simulink library "SpikingLib"  (Simulink 7.5)
settings: Solver=ode45  SolverMode=SingleTasking  StartTime=0.0  StopTime=10.0  RelTol=1e-3
undefined symbols (not defined in the file or in its folder): windowDuration
libraries: SpikingLib x13, simulink x3
settings Model: Creator=jpalma  LastModifiedBy=jpalma

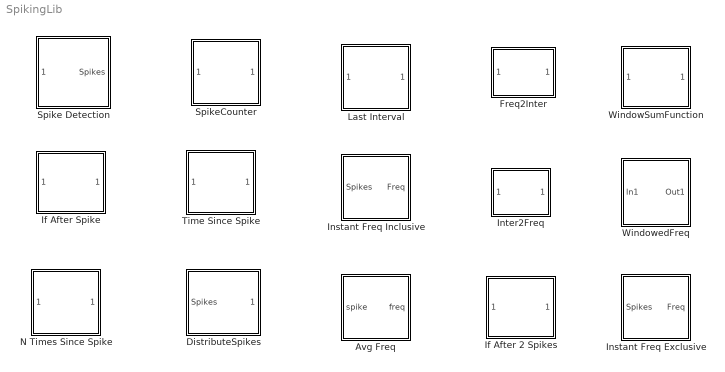
== system SpikingLib ==
  Avg Freq : Subsystem
      mask Description: Author: Jesse Palma
      mask Help: Author: Jesse Palma
      mask Display: image(imread('../Libs/icons/AvgFreq.jpg'),'center');
  DistributeSpikes : Subsystem  mask{numChannels=3}
      mask prompts: numChannels "Number of Channels"
      mask help:
      | Does not work with vectors of spike trains.
      |
      | Author: Jesse Palma
      mask Help: Author: Jesse Palma
      mask Display: image(imread('../Libs/icons/DistribSpikes.jpg'),'center');
  Freq2Inter : Subsystem
      mask Description: Author: Jesse Palma
      mask Help: Author: Jesse Palma
      mask Display: image(imread('../Libs/icons/FreqInter.jpg'),'center');
  If After 2 Spikes : Subsystem
      mask Description:
      | Are we after the second spike?
      | 
      | With an input vector of spike trains, this produces a vector of booleans of whether 2 spikes have arrived.
      | 
      | Author: Jesse Palma
      mask Help: Author: Jesse Palma
      mask Display: image(imread('../Libs/icons/IfAfterSpike.jpg'), 'center');
  If After Spike : Subsystem
      mask Description:
      | Are we after the first spike?
      | 
      | With an input vector of spike trains, this produces a vector of booleans of whether first spike has arrived.
      | 
      | Author: Jesse Palma
      mask Help: Author: Jesse Palma
      mask Display: image(imread('../Libs/icons/IfAfterSpike.jpg'), 'center');
  Instant Freq Exclusive : Subsystem
      mask Description:
      | Calculates frequency as 1 over the last interspike interval.
      | Frequency therefore isn't calculated until after the 2nd spike.
      | 
      | Author: Jesse Palma
      mask Help:
      | Calculates frequency as 1 over the last interspike interval.
      | Frequency therefore isn't calculated until after the 2nd spike.
      | 
      | Author: Jesse Palma
      mask Display: image(imread('../Libs/icons/InstantFreq.jpg'),'center');
  Instant Freq Inclusive : Subsystem
      mask Description:
      | Calculates frequency as 1 over the last interspike interval or the simulation time over first spike.
      | 
      | Author: Jesse Palma
      mask Help:
      | Calculates frequency as 1 over the last interspike interval or the simulation time over first spike.
      | 
      | Author: Jesse Palma
      mask Display: image(imread('../Libs/icons/InstantFreq.jpg'),'center');
  Inter2Freq : Subsystem
      mask Description: Author: Jesse Palma
      mask Help: Author: Jesse Palma
      mask Display: image(imread('../Libs/icons/InterFreq.jpg'),'center');
  Last Interval : Subsystem
      mask Description:
      | How long was the last interval?
      | 
      | With an input vector of spike trains, this produces a vector of last interspike interval durations.
      | 
      | Author: Jesse Palma
      mask Help: Author: Jesse Palma
      mask Display: image(imread('../Libs/icons/LastInterval.jpg'),'center');
  N Times Since Spike : Subsystem  mask{spikesMemory=10}
      mask prompts: spikesMemory "Size of Spikes Memory"
      mask help:
      | Does not work with vectors of spike trains.
      |
      | Author: Jesse Palma
      mask Help: Author: Jesse Palma
      mask Display: image(imread('../Libs/icons/NTimeSinceSpike.jpg'),'center');
  Spike Detection : Subsystem  mask{SpikeVoltageThreshold=10}
      mask prompts: SpikeVoltageThreshold "Spike Voltage Threshold"
      mask help: Author: Jesse Palma
      mask Help: Author: Jesse Palma
      mask Display: image(imread('../Libs/icons/SpikeDetection.jpg'),'center');
  SpikeCounter : Subsystem
      mask Description:
      | How many spikes so far?
      | 
      | With an input vector of spike trains, this produces a vector of the number of spikes arrived.
      | 
      | Author: Jesse Palma
      mask Help: Author: Jesse Palma
      mask Display: image(imread('../Libs/icons/SpikeCounter.jpg'),'center');
  Time Since Spike : Subsystem
      mask Description:
      | How long since the last spike?
      | 
      | With an input vector of spike trains, this produces a vector of times since the last spike arrived.
      | 
      | Author: Jesse Palma
      mask Help: Author: Jesse Palma
      mask Display: image(imread('../Libs/icons/TimeSinceSpike.jpg'),'center');
  WindowSumFunction : Subsystem  mask{windowDuration=windowDuration}
      mask prompts: windowDuration "Window Duration"
      mask help: Author: Jesse Palma
      mask Help: Author: Jesse Palma
      mask Display: image(imread('../Libs/icons/SquareWave.jpg'),'center');
  WindowedFreq : Subsystem  mask{windowDuration=60, spikesMemory=15}
      mask prompts: windowDuration "Window Duration"; spikesMemory "Max Number of Spikes Stored"
      mask help:
      | Note:
      |   maxFreq = spikesStored*1000/windowDuration
      |   freqPrecision = 1000/windowDuration
      | e.g. Defaults
      |   maxFreq = 15*1000/60 = 250
      |   freqPrecision = 1000/60 = 18
      |
      | Does not work with vectors of spike trains.
      |
      | Author: Jesse Palma
      mask Help: Author: Jesse Palma
      mask Display: image(imread('../Libs/icons/WindFreq.jpg'),'center');

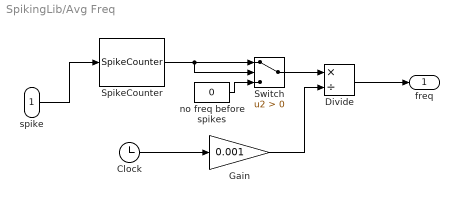
== system SpikingLib/Avg Freq ==
  spike : Inport
  Clock : Clock
      settings: Decimation=10
  Divide : Product  Inputs=*/
  Gain : Gain  Gain=0.001
  SpikeCounter : SpikingLib/SpikeCounter  SystemSampleTime=-1
  Switch : Switch  Criteria=u2 > Threshold
  no freq before spikes : Constant  Value=0
  freq : Outport
  wires:
  Divide/1 -> freq/1
  spike/1 -> SpikeCounter/1
  Clock/1 -> Gain/1
  Gain/1 -> Divide/2
  no freq before spikes/1 -> Switch/3
  Switch/1 -> Divide/1
  SpikeCounter/1 -> Switch/2, Switch/1

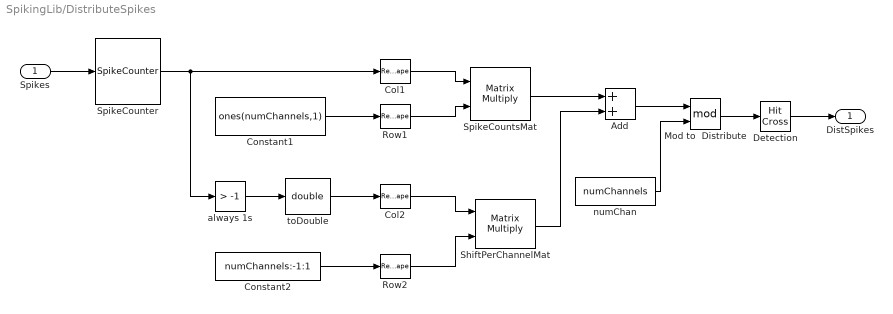
== system SpikingLib/DistributeSpikes ==
  Spikes : Inport
  Add : Sum
  Col1 : Reshape  OutputDimensionality=Column vector (2-D)
  Col2 : Reshape  OutputDimensionality=Column vector (2-D)
  Constant1 : Constant  Value=ones(numChannels,1)
  Constant2 : Constant  Value=numChannels:-1:1
  Detection : HitCross  HitCrossingDirection=rising
  Mod to  Distribute : Math  Operator=mod  SaturateOnIntegerOverflow=on
  Row1 : Reshape  OutputDimensionality=Row vector (2-D)
  Row2 : Reshape  OutputDimensionality=Row vector (2-D)
  ShiftPerChannelMat : Product  Multiplication=Matrix(*)  RndMeth=Zero
  SpikeCounter : SpikingLib/SpikeCounter  SystemSampleTime=-1
  SpikeCountsMat : Product  Multiplication=Matrix(*)  RndMeth=Zero
  always 1s : simulink/Logic and Bit Operations/Compare To Constant  SystemSampleTime=-1  relop=>  const=-1  LogicOutDataTypeMode=uint8  ZeroCross=off
  numChan : Constant  Value=numChannels
  toDouble : DataTypeConversion  OutDataTypeMode=double  OutDataTypeStr=double
  DistSpikes : Outport
  wires:
  SpikeCounter/1 -> always 1s/1, Col1/1
  numChan/1 -> Mod to  Distribute/2
  Mod to  Distribute/1 -> Detection/1
  Col1/1 -> SpikeCountsMat/1
  Constant1/1 -> Row1/1
  Constant2/1 -> Row2/1
  always 1s/1 -> toDouble/1
  toDouble/1 -> Col2/1
  Row2/1 -> ShiftPerChannelMat/2
  SpikeCountsMat/1 -> Add/1
  ShiftPerChannelMat/1 -> Add/2
  Add/1 -> Mod to  Distribute/1
  Spikes/1 -> SpikeCounter/1
  Detection/1 -> DistSpikes/1
  Col2/1 -> ShiftPerChannelMat/1
  Row1/1 -> SpikeCountsMat/2

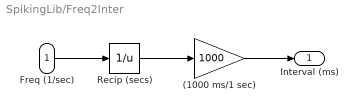
== system SpikingLib/Freq2Inter ==
  Freq (1/sec) : Inport
  (1000 ms/1 sec) : Gain  Gain=1000
  Recip (secs) : Math  Operator=reciprocal  SaturateOnIntegerOverflow=on
  Interval (ms) : Outport
  wires:
  (1000 ms/1 sec)/1 -> Interval (ms)/1
  Freq (1/sec)/1 -> Recip (secs)/1
  Recip (secs)/1 -> (1000 ms/1 sec)/1

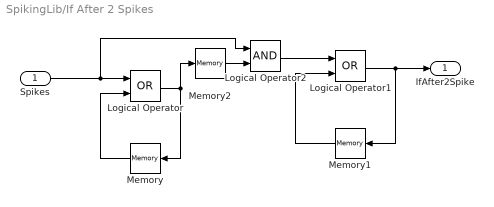
== system SpikingLib/If After 2 Spikes ==
  Spikes : Inport
  Logical Operator : Logic  Operator=OR  AllPortsSameDT=off  OutDataTypeMode=boolean  OutDataTypeStr=boolean
  Logical Operator1 : Logic  Operator=OR  AllPortsSameDT=off  OutDataTypeMode=boolean  OutDataTypeStr=boolean
  Logical Operator2 : Logic  AllPortsSameDT=off  OutDataTypeMode=boolean  OutDataTypeStr=boolean
  Memory : Memory
  Memory1 : Memory
  Memory2 : Memory
  IfAfter2Spike : Outport
  wires:
  Logical Operator/1 -> Memory/1, Memory2/1
  Memory/1 -> Logical Operator/2
  Spikes/1 -> Logical Operator/1, Logical Operator2/1
  Logical Operator1/1 -> IfAfter2Spike/1, Memory1/1
  Memory1/1 -> Logical Operator1/2
  Logical Operator2/1 -> Logical Operator1/1
  Memory2/1 -> Logical Operator2/2

== system SpikingLib/If After Spike ==
  Spikes : Inport
  Logical Operator : Logic  Operator=OR  AllPortsSameDT=off  OutDataTypeMode=boolean  OutDataTypeStr=boolean
  Memory : Memory
  IfAfterSpike : Outport
  wires:
  Memory/1 -> Logical Operator/2
  Spikes/1 -> Logical Operator/1
  Logical Operator/1 -> Memory/1, IfAfterSpike/1

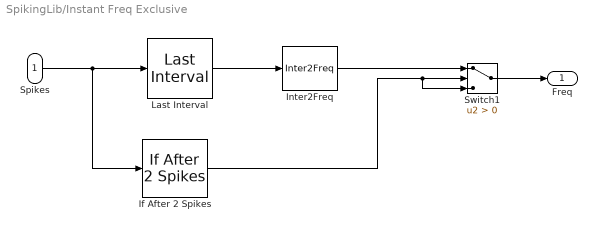
== system SpikingLib/Instant Freq Exclusive ==
  Spikes : Inport
  If After 2 Spikes : SpikingLib/If After 2 Spikes  SystemSampleTime=-1
  Inter2Freq : SpikingLib/Inter2Freq  SystemSampleTime=-1
  Last Interval : SpikingLib/Last Interval  SystemSampleTime=-1
  Switch1 : Switch  Criteria=u2 > Threshold
  Freq : Outport
  wires:
  Last Interval/1 -> Inter2Freq/1
  Spikes/1 -> Last Interval/1, If After 2 Spikes/1
  Inter2Freq/1 -> Switch1/1
  If After 2 Spikes/1 -> Switch1/2, Switch1/3
  Switch1/1 -> Freq/1

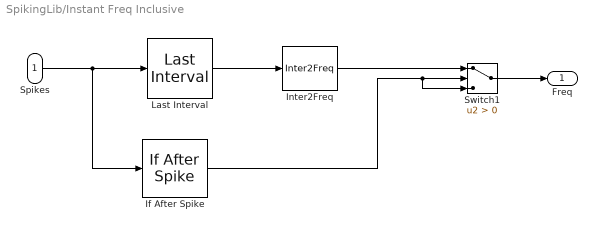
== system SpikingLib/Instant Freq Inclusive ==
  Spikes : Inport
  If After Spike : SpikingLib/If After Spike  SystemSampleTime=-1
  Inter2Freq : SpikingLib/Inter2Freq  SystemSampleTime=-1
  Last Interval : SpikingLib/Last Interval  SystemSampleTime=-1
  Switch1 : Switch  Criteria=u2 > Threshold
  Freq : Outport
  wires:
  Switch1/1 -> Freq/1
  If After Spike/1 -> Switch1/3, Switch1/2
  Inter2Freq/1 -> Switch1/1
  Spikes/1 -> If After Spike/1, Last Interval/1
  Last Interval/1 -> Inter2Freq/1

== system SpikingLib/Inter2Freq ==
  Interval (ms) : Inport
  (1000 ms/1 sec) : Gain  Gain=1000
  Recip (1/ms) : Math  Operator=reciprocal  SaturateOnIntegerOverflow=on
  Freq (1/sec) : Outport
  wires:
  Interval (ms)/1 -> Recip (1/ms)/1
  Recip (1/ms)/1 -> (1000 ms/1 sec)/1
  (1000 ms/1 sec)/1 -> Freq (1/sec)/1

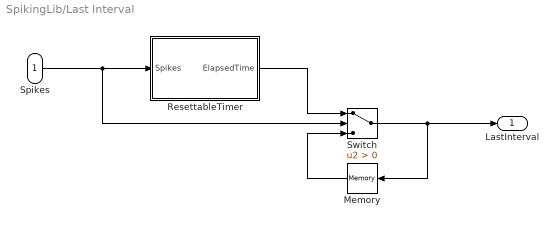
== system SpikingLib/Last Interval ==
  Spikes : Inport
  Memory : Memory
  ResettableTimer : Subsystem
  Switch : Switch  Criteria=u2 > Threshold
  LastInterval : Outport
  wires:
  Switch/1 -> LastInterval/1, Memory/1
  Memory/1 -> Switch/3
  Spikes/1 -> Switch/2, ResettableTimer/1(Spikes)
  ResettableTimer/1(ElapsedTime) -> Switch/1

== system SpikingLib/N Times Since Spike ==
  Spikes : Inport
  DistributeSpikes : SpikingLib/DistributeSpikes  SystemSampleTime=-1  numChannels=spikesMemory
  Time Since Spike : SpikingLib/Time Since Spike  SystemSampleTime=-1
  TimesSinceSpike : Outport
  wires:
  Spikes/1 -> DistributeSpikes/1
  DistributeSpikes/1 -> Time Since Spike/1
  Time Since Spike/1 -> TimesSinceSpike/1

== system SpikingLib/Spike Detection ==
  Voltage : Inport
  Spike Detection : HitCross  HitCrossingOffset=SpikeVoltageThreshold  HitCrossingDirection=rising
  Spikes : Outport
  wires:
  Voltage/1 -> Spike Detection/1
  Spike Detection/1 -> Spikes/1

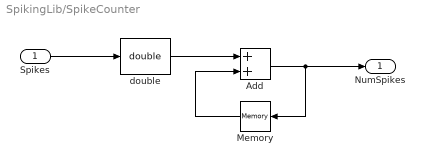
== system SpikingLib/SpikeCounter ==
  Spikes : Inport
  Add : Sum
  Memory : Memory
  double : DataTypeConversion  OutDataTypeMode=double  OutDataTypeStr=double
  NumSpikes : Outport
  wires:
  double/1 -> Add/1
  Spikes/1 -> double/1
  Memory/1 -> Add/2
  Add/1 -> Memory/1, NumSpikes/1

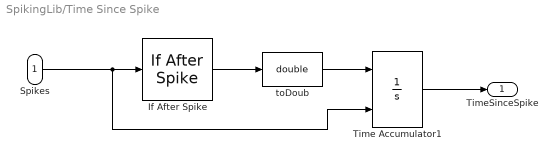
== system SpikingLib/Time Since Spike ==
  Spikes : Inport
  If After Spike : SpikingLib/If After Spike  SystemSampleTime=-1
  Time Accumulator1 : Integrator  ExternalReset=rising
  toDoub : DataTypeConversion  OutDataTypeMode=double  OutDataTypeStr=double
  TimeSinceSpike : Outport
  wires:
  Time Accumulator1/1 -> TimeSinceSpike/1
  toDoub/1 -> Time Accumulator1/1
  If After Spike/1 -> toDoub/1
  Spikes/1 -> Time Accumulator1/2, If After Spike/1

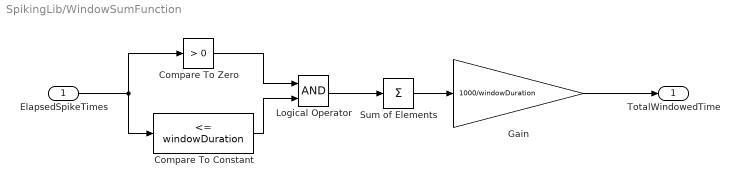
== system SpikingLib/WindowSumFunction ==
  ElapsedSpikeTimes : Inport
  Compare To Constant : simulink/Logic and Bit Operations/Compare To Constant  SystemSampleTime=-1  relop=<=  const=windowDuration  LogicOutDataTypeMode=uint8  ZeroCross=off
  Compare To Zero : simulink/Logic and Bit Operations/Compare To Zero  SystemSampleTime=-1  relop=>  LogicOutDataTypeMode=uint8  ZeroCross=off
  Gain : Gain  Gain=1000/windowDuration
  Logical Operator : Logic  AllPortsSameDT=off  OutDataTypeMode=boolean  OutDataTypeStr=boolean
  Sum of Elements : Sum  Inputs=+  CollapseMode=Specified dimension  CollapseDim=2
  TotalWindowedTime : Outport
  wires:
  ElapsedSpikeTimes/1 -> Compare To Constant/1, Compare To Zero/1
  Sum of Elements/1 -> Gain/1
  Logical Operator/1 -> Sum of Elements/1
  Compare To Zero/1 -> Logical Operator/1
  Compare To Constant/1 -> Logical Operator/2
  Gain/1 -> TotalWindowedTime/1

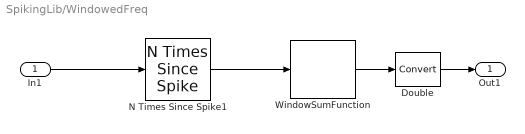
== system SpikingLib/WindowedFreq ==
  In1 : Inport
  Double : DataTypeConversion
  N Times Since Spike1 : SpikingLib/N Times Since Spike  SystemSampleTime=-1  spikesMemory=spikesMemory
  WindowSumFunction : SpikingLib/WindowSumFunction  SystemSampleTime=-1  windowDuration=windowDuration
  Out1 : Outport
  wires:
  WindowSumFunction/1 -> Double/1
  In1/1 -> N Times Since Spike1/1
  N Times Since Spike1/1 -> WindowSumFunction/1
  Double/1 -> Out1/1

== system SpikingLib/Last Interval/ResettableTimer ==
  Spikes : Inport
  RateOfTime : Constant
  Time Accumulator : Integrator  ExternalReset=falling
  ElapsedTime : Outport  InitialOutput=0
  wires:
  Time Accumulator/1 -> ElapsedTime/1
  Spikes/1 -> Time Accumulator/2
  RateOfTime/1 -> Time Accumulator/1
